simulink library "ctrlAllocMatrixLE_cl"  (R2018b)
settings: Solver=VariableStepAuto  StartTime=0.0  StopTime=10.0  RelTol=1e-3
undefined symbols (not defined in the file): aeroStruct, fluidDensity, pathCtrl, vhcl
libraries: vrlib x3, dspstat3 x2, vectorNormalizer_ul x2, eulAng2RotMat_ul x1, linearLeastSqrs_ul x1, dynamicPressure_ul x1, alphaBetaLE_ul x1, localApparentWind_ul x1, rotateAboutVec x1
settings Model: Creator=mcobb  LastModifiedBy=jldanie5

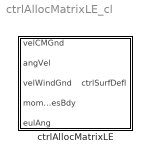
== system ctrlAllocMatrixLE_cl ==
  ctrlAllocMatrixLE : Subsystem  mask{aeroStruct=aeroStruct, fluidDensity=fluidDensity, ctrlUpMax=pathCtrl.controlSigMax.upperLimit.Value, ctrlDnMax=pathCtrl.controlSigMax.lowerLimit.Value}
      mask prompts: aeroStruct "Aerodynamic surface structure"; fluidDensity "Fluid density"; ctrlUpMax "Max Up Ctrl Surf Defl"; ctrlDnMax "Max Down Ctrl Surf Defl"
      settings: MinAlgLoopOccurrences=on
      mask TypeOptions aeroStruct: momentComponentVector/aeroStruct
      mask TypeOptions fluidDensity: momentComponentVector/fluidDensity

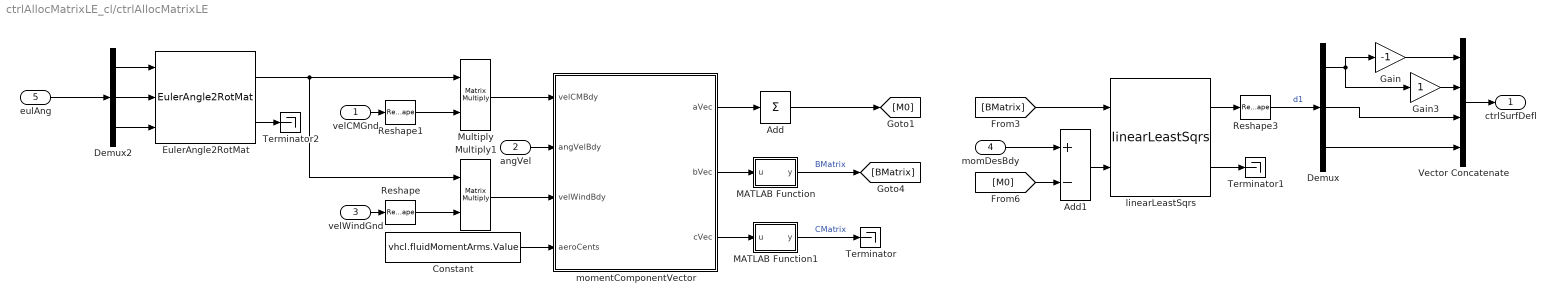
== system ctrlAllocMatrixLE_cl/ctrlAllocMatrixLE ==
  velCMGnd : Inport
  angVel : Inport  Port=2
  velWindGnd : Inport  Port=3
  momDesBdy : Inport  Port=4
  eulAng : Inport  Port=5
  Add : Sum  Inputs=+  CollapseMode=Specified dimension  CollapseDim=2
  Add1 : Sum  Inputs=+-
  Constant : Constant  Value=vhcl.fluidMomentArms.Value
  Demux : Demux  Outputs=3
  Demux2 : Demux  Outputs=3
  EulerAngle2RotMat : eulAng2RotMat_ul/EulerAngle2RotMat  SystemSampleTime=-1
  Gain : Gain  Gain=-1
  Gain3 : Gain
  MATLAB Function : MATLAB Function  TreatAsAtomicUnit=on
  MATLAB Function1 : MATLAB Function  TreatAsAtomicUnit=on
  Multiply : Product  Multiplication=Matrix(*)
  Multiply1 : Product  Multiplication=Matrix(*)
  Reshape : Reshape  OutputDimensionality=Column vector (2-D)
  Reshape1 : Reshape  OutputDimensionality=Column vector (2-D)
  Reshape3 : Reshape
  Terminator : Terminator
  Terminator1 : Terminator
  Terminator2 : Terminator
  Vector Concatenate : Concatenate  NumInputs=4
  linearLeastSqrs : linearLeastSqrs_ul/linearLeastSqrs  SystemSampleTime=-1
  momentComponentVector : Subsystem  mask{aeroStruct=aeroStruct, fluidDensity=fluidDensity}
      mask prompts: aeroStruct "Aerodynamic surface structure"; fluidDensity "Fluid density"
      mask help:
      | Input must be an 1×N struct array with fields:
      |     refArea
      |     aeroCentPosVec
      |     spanUnitVec
      |     chordUnitVec
      |     CL
      |     CD
      |     alpha
      |     GainCL
      |     GainCD
      |
      | where N is the number of aerodynamic surfaces
  ctrlSurfDefl : Outport
  wires:
  Demux2/2 -> EulerAngle2RotMat/2
  eulAng/1 -> Demux2/1
  velWindGnd/1 -> Reshape/1
  EulerAngle2RotMat/2 -> Terminator2/1
  velCMGnd/1 -> Reshape1/1
  Multiply/1 -> momentComponentVector/1(velCMBdy)
  Reshape/1 -> Multiply1/2
  Demux2/1 -> EulerAngle2RotMat/1
  Reshape1/1 -> Multiply/2
  Demux2/3 -> EulerAngle2RotMat/3
  Multiply1/1 -> momentComponentVector/3(velWindBdy)
  EulerAngle2RotMat/1 -> Multiply1/1, Multiply/1
  Gain3/1 -> Vector Concatenate/2
  Vector Concatenate/1 -> ctrlSurfDefl/1
  Demux/3 -> Vector Concatenate/4
  Demux/2 -> Vector Concatenate/3
  Demux/1 -> Gain/1, Gain3/1
  Gain/1 -> Vector Concatenate/1
  [BMatrix] -> linearLeastSqrs/1
  linearLeastSqrs/1 -> Reshape3/1
  momDesBdy/1 -> Add1/1
  MATLAB Function1/1(y) -> Terminator/1  "CMatrix"
  linearLeastSqrs/2 -> Terminator1/1
  momentComponentVector/2(bVec) -> MATLAB Function/1(u)
  Reshape3/1 -> Demux/1  "d1"
  MATLAB Function/1(y) -> [BMatrix]  "BMatrix"
  Add1/1 -> linearLeastSqrs/2
  [M0] -> Add1/2
  Add/1 -> [M0]
  momentComponentVector/3(cVec) -> MATLAB Function1/1(u)
  momentComponentVector/1(aVec) -> Add/1
  angVel/1 -> momentComponentVector/2(angVelBdy)
  Constant/1 -> momentComponentVector/4(aeroCents)

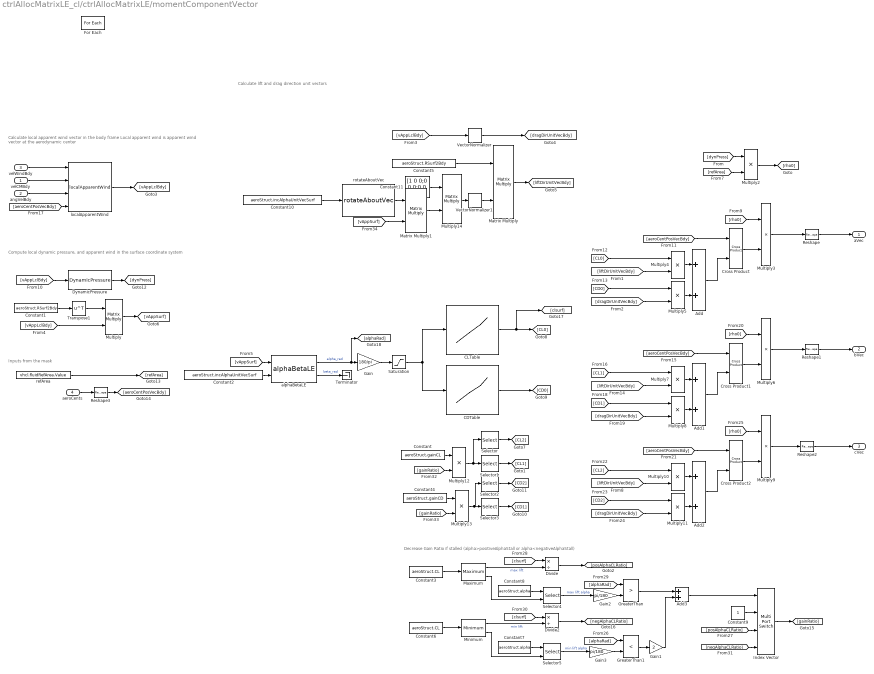
== system ctrlAllocMatrixLE_cl/ctrlAllocMatrixLE/momentComponentVector ==
  note: Decrease Gain Ratio if stalled (alpha>positiveAlphaStall or alpha<negativeAlphaStall)
  note: Calculate local apparent wind vector in the body frame
      | Local apparent wind is apparent wind vector at the aerodynamic center
  note: Calculate lift and drag direction unit vectors
  note: Inputs from the mask
  note: Compute local dynamic pressure,
      | and apparent wind in the surface coordinate system
  velCMBdy : Inport
  angVelBdy : Inport  Port=2
  velWindBdy : Inport  Port=3
  aeroCents : Inport  Port=4  Partition=on  PartitionDimension=2  PartitionWidth=1  PartitionOffset=0
  Add{,1..3} (4 alike) : Sum
  CDTable : Lookup_n-D  NumberOfTableDimensions=1  LookupTableObject=CLTable  BreakpointsForDimension1=aeroStruct.alpha  Table=aeroStruct.CD  ExtrapMethod=Clip  UseLastTableValue=on  InternalRulePriority=Speed  RndMeth=Simplest  InputSameDT=on
  CLTable : Lookup_n-D  NumberOfTableDimensions=1  LookupTableObject=CLTable  BreakpointsForDimension1=aeroStruct.alpha  Table=aeroStruct.CL  ExtrapMethod=Clip  UseLastTableValue=on  InternalRulePriority=Speed  RndMeth=Simplest  InputSameDT=on
  Constant : Constant  Value=aeroStruct.gainCL
  Constant1 : Constant  Value=aeroStruct.RSurf2Bdy
  Constant10 : Constant  Value=aeroStruct.incAlphaUnitVecSurf
  Constant11 : Constant  Value=[1 0 0;0 0 0;0 0 1]
  Constant2 : Constant  Value=aeroStruct.incAlphaUnitVecSurf
  Constant3 : Constant  Value=aeroStruct.CL
  Constant4 : Constant  Value=aeroStruct.gainCD
  Constant5 : Constant  Value=aeroStruct.RSurf2Bdy
  Constant6 : Constant  Value=aeroStruct.CL
  Constant7 : Constant  Value=aeroStruct.alpha
  Constant8 : Constant  Value=aeroStruct.alpha
  Constant9 : Constant
  Cross Product : vrlib/Utilities/Cross Product
      settings: SourceProductBaseCode=VR
  Cross Product1 : vrlib/Utilities/Cross Product
      settings: SourceProductBaseCode=VR
  Cross Product2 : vrlib/Utilities/Cross Product
      settings: SourceProductBaseCode=VR
  Divide : Product  Inputs=*/
  Divide2 : Product  Inputs=*/
  DynamicPressure : dynamicPressure_ul/DynamicPressure  rho=fluidDensity
  For Each : ForEach  DisableCoverage=on  IterateSubsysMaskParameter=on,off  SubsysMaskParameterIterationDimension=2,1  IndexMode=One-based
  Gain : Gain  Gain=180/pi
  Gain1 : Gain  Gain=2
  Gain2 : Gain  Gain=pi/180
  Gain3 : Gain  Gain=pi/180
  GreaterThan : RelationalOperator  Operator=>  OutDataTypeStr=boolean  RndMeth=Simplest
  GreaterThan1 : RelationalOperator  Operator=<  OutDataTypeStr=boolean  RndMeth=Simplest
  Index Vector : MultiPortSwitch  DataPortOrder=Zero-based contiguous  zeroidx=on
  Matrix Multiply : Product  Multiplication=Matrix(*)
  Matrix Multiply1 : Product  Multiplication=Matrix(*)
  Maximum : dspstat3/Maximum  operation=maximum  fcn=Value and Index  indexBase=One  operateOver=Each column  Dimension=1  InputProcessing=Columns as channels (frame based)  reset=None  roiEnable=off  roiType=Rectangles  roiPortion=Entire ROI  roiOutput=Individual statistics for each ROI  roiFlag=off  roundingMode=Floor  overflowMode=off  accumDataTypeStr=Inherit: Same as product output  accumLastDataTypeStr=Inherit: Same as product output
  Minimum : dspstat3/Minimum  operation=minimum  fcn=Value and Index  indexBase=One  operateOver=Each column  Dimension=1  InputProcessing=Columns as channels (frame based)  reset=None  roiEnable=off  roiType=Rectangles  roiPortion=Entire ROI  roiOutput=Individual statistics for each ROI  roiFlag=off  roundingMode=Floor  overflowMode=off
      settings: SourceProductName=DSP System Toolbox  SourceProductBaseCode=DS
  Multiply : Product  Multiplication=Matrix(*)
  Multiply{2..13} (12 alike) : Product
  Multiply14 : Product  Multiplication=Matrix(*)
  Reshape{,1..3} (4 alike) : Reshape  OutputDimensionality=Column vector (2-D)
  Saturation : Saturate  UpperLimit=90  LowerLimit=-90
  Selector : Selector  InputPortWidth=3  IndexOptions=Index vector (dialog)  Indices=1  OutputSizes=1
  Selector1 : Selector  InputPortWidth=3  IndexOptions=Index vector (dialog)  Indices=2  OutputSizes=1
  Selector2 : Selector  InputPortWidth=3  IndexOptions=Index vector (dialog)  Indices=1  OutputSizes=1
  Selector3 : Selector  InputPortWidth=3  IndexOptions=Index vector (dialog)  Indices=2  OutputSizes=1
  Selector4 : Selector  InputPortWidth=length(vhcl.portWing.alpha.Value)  IndexOptions=Index vector (port)  Indices=[1 3]  OutputSizes=1
  Selector5 : Selector  InputPortWidth=length(vhcl.portWing.alpha.Value)  IndexOptions=Index vector (port)  Indices=[1 3]  OutputSizes=1
  Terminator : Terminator
  Transpose1 : Math  Operator=transpose  SaturateOnIntegerOverflow=on
  "VectorNormalizer " : vectorNormalizer_ul/VectorNormalizer   SystemSampleTime=-1
  VectorNormalizer1 : vectorNormalizer_ul/VectorNormalizer   SystemSampleTime=-1
  alphaBetaLE : alphaBetaLE_ul/alphaBetaLE  SystemSampleTime=-1
  localApparentWind : localApparentWind_ul/localApparentWind  SystemSampleTime=-1
  refArea : Constant  Value=vhcl.fluidRefArea.Value
  rotateAboutVec : rotateAboutVec/rotateAboutVec  ang=90
  aVec : Outport  PortDimensions=[3 1]  ConcatenationDimension=2
  bVec : Outport  Port=2  PortDimensions=[3 1]  ConcatenationDimension=2
  cVec : Outport  Port=3  PortDimensions=[3 1]  ConcatenationDimension=2
  wires:
  Gain3/1 -> GreaterThan1/2
  Gain2/1 -> GreaterThan/2
  [gainRatio] -> Multiply13/2
  Constant4/1 -> Multiply13/1
  Multiply13/1 -> Selector3/1, Selector2/1
  Multiply12/1 -> Selector1/1, Selector/1
  [gainRatio] -> Multiply12/2
  Constant/1 -> Multiply12/1
  Divide2/1 -> [negAlphaCLRatio]
  Divide/1 -> [posAlphaCLRatio]
  GreaterThan/1 -> Add3/1
  Selector5/1 -> Gain3/1  "min lift alpha"
  [alphaRad] -> GreaterThan1/1
  Constant6/1 -> Minimum/1
  Gain1/1 -> Add3/2
  [posAlphaCLRatio] -> Index Vector/3
  Constant3/1 -> Maximum/1
  Constant7/1 -> Selector5/1
  Constant9/1 -> Index Vector/2
  Constant8/1 -> Selector4/1
  Maximum/1 -> Divide/2  "max lift"
  [negAlphaCLRatio] -> Index Vector/4
  Index Vector/1 -> [gainRatio]
  [alphaRad] -> GreaterThan/1
  GreaterThan1/1 -> Gain1/1
  Add3/1 -> Index Vector/1
  Selector4/1 -> Gain2/1  "max lift alpha"
  Minimum/1 -> Divide2/2  "min lift"
  Maximum/2 -> Selector4/2
  [clsurf] -> Divide/1
  Minimum/2 -> Selector5/2
  [clsurf] -> Divide2/1
  Reshape2/1 -> cVec/1
  Reshape1/1 -> bVec/1
  Reshape/1 -> aVec/1
  [CD2] -> Multiply11/1
  [CL2] -> Multiply10/1
  [liftDirUnitVecBdy] -> Multiply10/2
  [dragDirUnitVecBdy] -> Multiply11/2
  Multiply11/1 -> Add2/2
  Multiply10/1 -> Add2/1
  Add2/1 -> Cross Product2/2
  Multiply9/1 -> Reshape2/1
  [aeroCentPosVecBdy] -> Cross Product2/1
  Cross Product2/1 -> Multiply9/2
  [rho0] -> Multiply9/1
  [rho0] -> Multiply6/1
  Cross Product1/1 -> Multiply6/2
  [aeroCentPosVecBdy] -> Cross Product1/1
  Multiply6/1 -> Reshape1/1
  Add1/1 -> Cross Product1/2
  Multiply7/1 -> Add1/1
  Multiply8/1 -> Add1/2
  [dragDirUnitVecBdy] -> Multiply8/2
  [liftDirUnitVecBdy] -> Multiply7/2
  [CL1] -> Multiply7/1
  [CD1] -> Multiply8/1
  [CD0] -> Multiply5/1
  [CL0] -> Multiply4/1
  [liftDirUnitVecBdy] -> Multiply4/2
  [dragDirUnitVecBdy] -> Multiply5/2
  Multiply5/1 -> Add/2
  Multiply4/1 -> Add/1
  Add/1 -> Cross Product/2
  Multiply3/1 -> Reshape/1
  [aeroCentPosVecBdy] -> Cross Product/1
  Cross Product/1 -> Multiply3/2
  [rho0] -> Multiply3/1
  Multiply2/1 -> [rho0]
  [refArea] -> Multiply2/2
  [dynPress] -> Multiply2/1
  Selector3/1 -> [CD1]
  Selector2/1 -> [CD2]
  Selector/1 -> [CL2]
  Selector1/1 -> [CL1]
  Saturation/1 -> CLTable/1, CDTable/1
  CLTable/1 -> [CL0], [clsurf]
  Gain/1 -> Saturation/1
  localApparentWind/1 -> [vAppLclBdy]
  [aeroCentPosVecBdy] -> localApparentWind/4
  angVelBdy/1 -> localApparentWind/3
  velCMBdy/1 -> localApparentWind/2
  alphaBetaLE/1 -> Gain/1, [alphaRad]  "alpha_rad"
  Reshape3/1 -> [aeroCentPosVecBdy]
  refArea/1 -> [refArea]
  aeroCents/1 -> Reshape3/1
  VectorNormalizer1/1 -> Matrix Multiply/2
  Constant5/1 -> Matrix Multiply/1
  Matrix Multiply/1 -> [liftDirUnitVecBdy]
  [vAppLclBdy] -> DynamicPressure/1
  DynamicPressure/1 -> [dynPress]
  CDTable/1 -> [CD0]
  alphaBetaLE/2 -> Terminator/1  "beta_rad"
  Multiply14/1 -> VectorNormalizer1/1
  [vAppSurf] -> alphaBetaLE/1
  Multiply/1 -> [vAppSurf]
  [vAppLclBdy] -> Multiply/2
  Constant1/1 -> Transpose1/1
  "VectorNormalizer "/1 -> [dragDirUnitVecBdy]
  [vAppLclBdy] -> "VectorNormalizer "/1
  velWindBdy/1 -> localApparentWind/1
  Constant11/1 -> Multiply14/1
  rotateAboutVec/1 -> Matrix Multiply1/1
  [vAppSurf] -> Matrix Multiply1/2
  Constant10/1 -> rotateAboutVec/1
  Matrix Multiply1/1 -> Multiply14/2
  Constant2/1 -> alphaBetaLE/2
  Transpose1/1 -> Multiply/1

== matlab function ctrlAllocMatrixLE_cl/ctrlAllocMatrixLE/MATLAB Function1 ==
  data: u input; y output
function y = fcn(u)
y = [-u(:,1)+u(:,2) u(:,3:end)];

== matlab function ctrlAllocMatrixLE_cl/ctrlAllocMatrixLE/MATLAB Function ==
  data: u input; y output
function y = fcn(u)
y = [-u(:,1)+u(:,2) u(:,3:end)];
